simulink model "q2_simulink"  (R2023b)
settings: Solver=VariableStepAuto  StartTime=0.0  StopTime=2  RelTol=1e-3
values from neighbouring files (symbols this model uses):
  A = [0, 1,      0;       0, -b/J,   K/J;       0, -K/L, -R/L;]    [lec7_dc_motor_control_example.m]    (also in lec7_example_11.m = [0 0 4 1; lec7_notes_example_11.m = [-1, 1, 0;       0,  1, 1;       0,  0, 2;]; mini_proj_1.m = [-8.8487 + (a-b)/5,     -0.0399,              -5.55 + (c+d)/; mini_proj_q1.m = [-8.8487 + (a-b)/5,     -0.0399,              -5.55 + (c+d)/)
  B = [0;       0;       1/L;]    [lec7_dc_motor_control_example.m]    (also in lec7_example_11.m = [-2 0; lec7_notes_example_11.m = [1, 1;       0, 0;       0, 1;]; mini_proj_1.m = [0.0564+(b)/(10+c),           0.0319;       0.0165-(c+d-5)/(; mini_proj_q1.m = [0.0564+(b)/(10+c),           0.0319)
  C = [1, 0, 0]    [lec7_dc_motor_control_example.m]    (also in lec7_notes_example_11.m = [1, 3, -1;      0, 1,  0;]; mini_proj_1.m = [-3.2988,           -2.1932+(10*c+d)/(100+5*a), 0.0370,  -0.; mini_proj_q1.m = [-3.2988,           -2.1932+(10*c+d)/(100+5*a), 0.0370,  -0.; mini_proj_q2.m = [-3.2988,           -2.1932+(10*c+d)/(100+5*a), 0.0370,  -0.)
  K = transpose(place(A, B, des_poles))    [lec7_dc_motor_control_example.m]    (also in lec7_example_11.m = K_bar * T; lec7_notes_example_11.m = K_bar * T; mini_proj_1.m = K_bar * T; mini_proj_q1.m = K_bar * T)
  x_0 = [0.5; -0.1; 0.3; -0.8;]    [mini_proj_1.m]    (also in mini_proj_q1.m; mini_proj_q2.m; q1_full.m; q1_params.m)
settings Model: Creator=john  LastModifiedBy=john

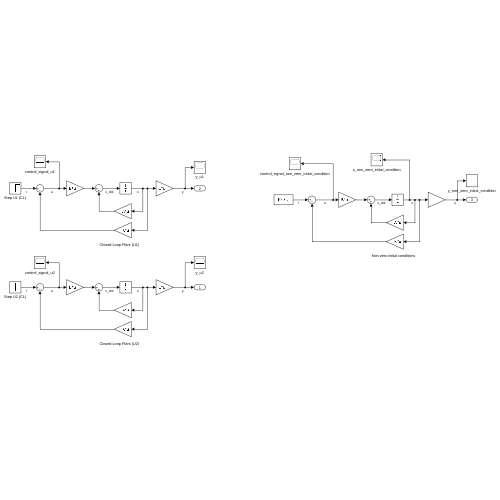
[thumbnail: Simulink's stored preview of the top-level diagram]
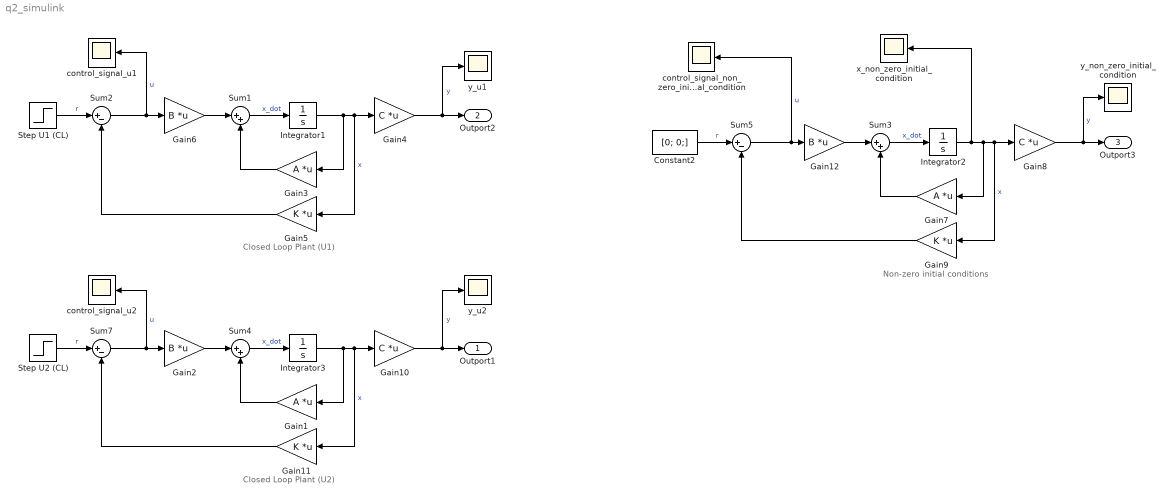
== system q2_simulink ==
  note: Closed Loop Plant (U1)
  note: Closed Loop Plant (U2)
  note: Non-zero initial conditions
  Constant2 : Constant  Value=[0; 0;]
  Gain1 : Gain  Gain=A  Multiplication=Matrix(K*u)
  Gain10 : Gain  Gain=C  Multiplication=Matrix(K*u)
  Gain11 : Gain  Gain=K  Multiplication=Matrix(K*u)
  Gain12 : Gain  Gain=B  Multiplication=Matrix(K*u)
  Gain2 : Gain  Gain=B  Multiplication=Matrix(K*u)
  Gain3 : Gain  Gain=A  Multiplication=Matrix(K*u)
  Gain4 : Gain  Gain=C  Multiplication=Matrix(K*u)
  Gain5 : Gain  Gain=K  Multiplication=Matrix(K*u)
  Gain6 : Gain  Gain=B  Multiplication=Matrix(K*u)
  Gain7 : Gain  Gain=A  Multiplication=Matrix(K*u)
  Gain8 : Gain  Gain=C  Multiplication=Matrix(K*u)
  Gain9 : Gain  Gain=K  Multiplication=Matrix(K*u)
  Integrator1 : Integrator
  Integrator2 : Integrator  InitialCondition=x_0
  Integrator3 : Integrator
  Step U1 (CL) : Step  Time=0  Before=[0; 0;];  After=[1; 0;];  SampleTime=0
  Step U2 (CL) : Step  Time=0  Before=[0; 0;];  After=[0; 1;];  SampleTime=0
  Sum1 : Sum  Inputs=|++
  Sum2 : Sum  Inputs=|+-
  Sum3 : Sum  Inputs=|++
  Sum4 : Sum  Inputs=|++
  Sum5 : Sum  Inputs=|+-
  Sum7 : Sum  Inputs=|+-
  control_signal_non_zero_initial_condition : Scope
  control_signal_u1 : Scope
  control_signal_u2 : Scope
  x_non_zero_initial_condition : Scope
  y_non_zero_initial_condition : Scope
  y_u1 : Scope
  y_u2 : Scope
  Outport1 : Outport
  Outport2 : Outport  Port=2
  Outport3 : Outport  Port=3
  wires:
  Integrator1/1 -> Gain3/1, Gain5/1, Gain4/1  "x"
  Gain5/1 -> Sum2/2
  Step U2 (CL)/1 -> Sum7/1  "r"
  Gain10/1 -> y_u2/1, Outport1/1  "y"
  Gain1/1 -> Sum4/2
  Sum1/1 -> Integrator1/1  "x_dot"
  Integrator3/1 -> Gain1/1, Gain11/1, Gain10/1  "x"
  Gain11/1 -> Sum7/2
  Gain6/1 -> Sum1/1
  Sum2/1 -> control_signal_u1/1, Gain6/1  "u"
  Sum7/1 -> control_signal_u2/1, Gain2/1  "u"
  Gain4/1 -> y_u1/1, Outport2/1  "y"
  Gain2/1 -> Sum4/1
  Gain3/1 -> Sum1/2
  Step U1 (CL)/1 -> Sum2/1  "r"
  Sum4/1 -> Integrator3/1  "x_dot"
  Sum3/1 -> Integrator2/1  "x_dot"
  Sum5/1 -> control_signal_non_zero_initial_condition/1, Gain12/1  "u"
  Gain12/1 -> Sum3/1
  Gain8/1 -> y_non_zero_initial_condition/1, Outport3/1  "y"
  Integrator2/1 -> x_non_zero_initial_condition/1, Gain7/1, Gain9/1, Gain8/1  "x"
  Gain9/1 -> Sum5/2
  Gain7/1 -> Sum3/2
  Constant2/1 -> Sum5/1  "r"
